simulink model "EvPowertrainController3EMDualFront"  (R2023a)
settings: configuration reference "VehicleFixed10ms" (kept outside this file)
model workspace (MAT data in the model file):
  CtrlVcuCnstrntPnltyFctr = 10000000
  CtrlVcuEMTrqSplitGrid = 200
  CtrlVcuPwrDeltaPnlty = 2
  CtrlVcuTracPwrErrPnlty = 6
  CtrlVcuTrqVecBrkThresh = 0.01
  CtrlVcuTrqVecIGain = 0
  CtrlVcuTrqVecMinTrq = 50
  CtrlVcuTrqVecPGain = -2000
  CtrlVcuTrqVecSteerThresh = 0.349065850399
  CtrlVcuTrqVecVelThresh = 2.5
undefined symbols (not defined in the file): CtrlVcuEvChrgLmtBpt, CtrlVcuEvRegenBrkCutOff, CtrlVcuEvRegenBrkSpdBpt, CtrlVcuEvSocBpt, eff, PlntBrkActrBoreFrnt, PlntBrkFrntBias, PlntBrkKinFricCffFrnt, PlntBrkNumPadsFrnt, PlntBrkPadMeanRadiusFrnt, PlntBrkPrsFctr, PlntBrkRearBias, PlntDiffrntl2Eff, PlntDiffrntl2Ratio, PlntDiffrntlEff, PlntDiffrntlRatio, PlntEM1EffTbl, PlntEM1Spd, PlntEM1Trq, PlntEM1TrqEff, PlntEM2EffTbl, PlntEM2Spd, PlntEM2Trq, PlntEM2TrqEff, PlntEM3EffTbl, PlntEM3Spd, PlntEM3Trq, PlntEM3TrqEff, PlntEMWhlGearEffFL, PlntEMWhlGearEffRL, PlntEMWhlGearRatioFL, PlntEMWhlGearRatioRL, PlntTransEffSpdBpt, PlntTransEffTbl, PlntTransEffTempBpt, PlntTransEffTrqBpt, PlntTransGearNumVect, PlntTransGearRatioVect, PlntVehDstCGFrntAxl, PlntVehDstCGRearAxl, PlntWhlLdRadius
libraries: simulink x13, autolibutils x2, slpidlib x2
(part 2 of 5)

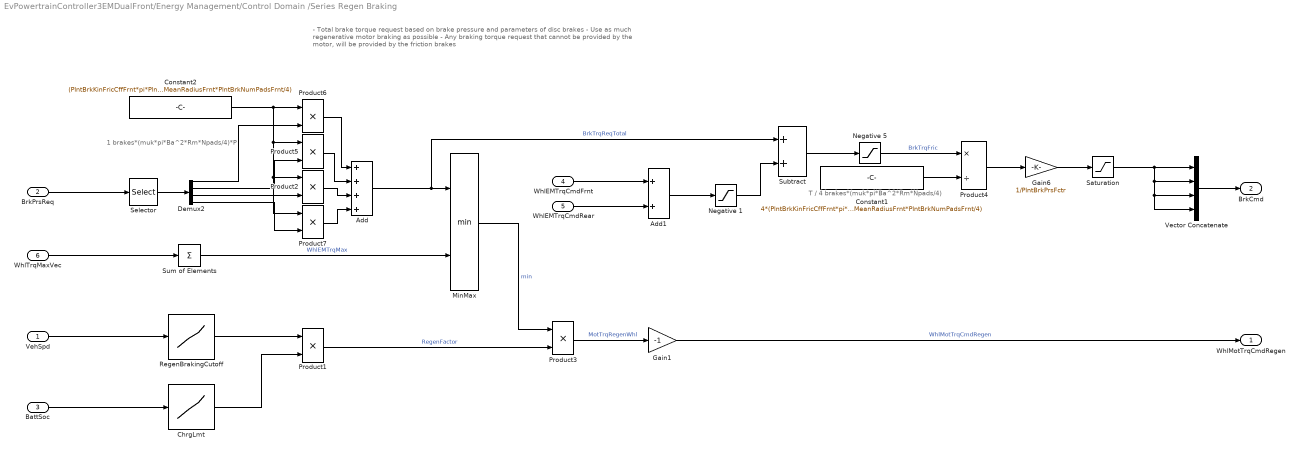
== system EvPowertrainController3EMDualFront/Energy Management/Control Domain /Series Regen Braking ==
  note: - Total brake torque request based on brake pressure and parameters of disc brakes
      | - Use as much regenerative motor braking as possible
      | - Any braking torque request that cannot be provided by the motor, will be provided by the friction brakes
  note: T / 4 brakes*(muk*pi*Ba^2*Rm*Npads/4)
  note: 1 brakes*(muk*pi*Ba^2*Rm*Npads/4)*P
  VehSpd : Inport
  "BrkPrsReq " : Inport  Port=2
  BattSoc : Inport  Port=3
  WhlEMTrqCmdFrnt : Inport  Port=4
  WhlEMTrqCmdRear : Inport  Port=5
  WhlTrqMaxVec : Inport  Port=6
  Add : Sum  Inputs=++++
  Add1 : Sum
  ChrgLmt : Lookup_n-D  NumberOfTableDimensions=1  BreakpointsForDimension1=CtrlVcuEvSocBpt  Table=CtrlVcuEvChrgLmtBpt  ExtrapMethod=Clip  UseLastTableValue=on  InternalRulePriority=Speed  RndMeth=Simplest
  Constant1 : Constant  Value=4*(PlntBrkKinFricCffFrnt*pi*PlntBrkActrBoreFrnt^2*PlntBrkPadMeanRadiusFrnt*PlntBrkNumPadsFrnt/4)
  Constant2 : Constant  Value=(PlntBrkKinFricCffFrnt*pi*PlntBrkActrBoreFrnt^2*PlntBrkPadMeanRadiusFrnt*PlntBrkNumPadsFrnt/4)
  Demux2 : Demux
  Gain1 : Gain  Gain=-1
  Gain6 : Gain  Gain=1/PlntBrkPrsFctr
  MinMax : MinMax  Inputs=2
  Negative 1 : Saturate  UpperLimit=0  LowerLimit=-inf
  Negative 5 : Saturate  UpperLimit=inf  LowerLimit=0
  Product{1..3,5..7} (6 alike) : Product
  Product4 : Product  Inputs=*/
  RegenBrakingCutoff : Lookup_n-D  NumberOfTableDimensions=1  BreakpointsForDimension1=CtrlVcuEvRegenBrkSpdBpt  Table=CtrlVcuEvRegenBrkCutOff  ExtrapMethod=Clip  UseLastTableValue=on  InternalRulePriority=Speed  RndMeth=Simplest
  Saturation : Saturate  UpperLimit=1  LowerLimit=0
  Selector : Selector  InputPortWidth=4  IndexOptions=Index vector (dialog)  Indices=[1 2 3 4]  OutputSizes=1
  Subtract : Sum
  Sum of Elements : Sum  Inputs=+
  Vector Concatenate : Concatenate  NumInputs=4
  " WhlMotTrqCmdRegen" : Outport  VectorParamsAs1DForOutWhenUnconnected=off
  " BrkCmd" : Outport  Port=2  VectorParamsAs1DForOutWhenUnconnected=off
  wires:
  Constant1/1 -> Product4/2
  MinMax/1 -> Product3/1  "min"
  ChrgLmt/1 -> Product1/2
  VehSpd/1 -> RegenBrakingCutoff/1
  RegenBrakingCutoff/1 -> Product1/1
  Product1/1 -> Product3/2  "RegenFactor"
  Subtract/1 -> Negative 5/1
  BattSoc/1 -> ChrgLmt/1
  Negative 5/1 -> Product4/1  "BrkTrqFric"
  Sum of Elements/1 -> MinMax/2  "WhlEMTrqMax"
  Demux2/2 -> Product5/2
  Demux2/1 -> Product6/2
  Selector/1 -> Demux2/1
  Product6/1 -> Add/1
  Product5/1 -> Add/2
  Add/1 -> Subtract/1, MinMax/1  "BrkTrqReqTotal"
  "BrkPrsReq "/1 -> Selector/1
  Vector Concatenate/1 -> " BrkCmd"/1
  Gain6/1 -> Saturation/1
  Product4/1 -> Gain6/1
  Saturation/1 -> Vector Concatenate/3, Vector Concatenate/4, Vector Concatenate/2, Vector Concatenate/1
  WhlTrqMaxVec/1 -> Sum of Elements/1
  Gain1/1 -> " WhlMotTrqCmdRegen"/1  "WhlMotTrqCmdRegen"
  Product3/1 -> Gain1/1  "MotTrqRegenWhl"
  Add1/1 -> Negative 1/1
  Negative 1/1 -> Subtract/2
  Product2/1 -> Add/3
  Product7/1 -> Add/4
  Demux2/3 -> Product2/2
  Demux2/4 -> Product7/2
  Constant2/1 -> Product7/1, Product2/1, Product5/1, Product6/1
  WhlEMTrqCmdFrnt/1 -> Add1/1
  WhlEMTrqCmdRear/1 -> Add1/2

== system EvPowertrainController3EMDualFront/Energy Management/Convert Whl to EMTrq Vector/2EM ==
  WhlEMTrqCmdFrnt : Inport
  WhlEMTrqCmdRear : Inport  Port=2
  EMAvgSpdVec : Inport  Port=3
  Diff Eta : Subsystem
  Diff Eta1 : Subsystem
  Divide1 : Product  Inputs=/*
  Divide2 : Product  Inputs=/*
  Gain1 : Gain  Gain=1/PlntDiffrntl2Ratio
  Gain3 : Gain  Gain=1/PlntDiffrntlRatio
  Selector : Selector  InputPortWidth=2  IndexOptions=Index vector (dialog)  Indices=[1]  OutputSizes=1
  Selector1 : Selector  InputPortWidth=2  IndexOptions=Index vector (dialog)  Indices=[2]  OutputSizes=1
  Unit Delay : UnitDelay  SampleTime=-1  HasFrameUpgradeWarning=on
  Unit Delay1 : UnitDelay  SampleTime=-1  HasFrameUpgradeWarning=on
  Vector Concatenate1 : Concatenate
  EMTrqCmd : Outport
  wires:
  WhlEMTrqCmdRear/1 -> Gain1/1
  Gain3/1 -> Divide2/2
  Divide2/1 -> Vector Concatenate1/1, Unit Delay/1
  WhlEMTrqCmdFrnt/1 -> Gain3/1
  Selector/1 -> Diff Eta/1(SpdIn)
  Unit Delay/1 -> Diff Eta/2(TrqIn)
  Diff Eta/1(eta) -> Divide2/1
  Diff Eta1/1(eta) -> Divide1/1
  Unit Delay1/1 -> Diff Eta1/2(TrqIn)
  Divide1/1 -> Unit Delay1/1, Vector Concatenate1/2
  Gain1/1 -> Divide1/2
  EMAvgSpdVec/1 -> Selector1/1, Selector/1
  Selector1/1 -> Diff Eta1/1(SpdIn)
  Vector Concatenate1/1 -> EMTrqCmd/1

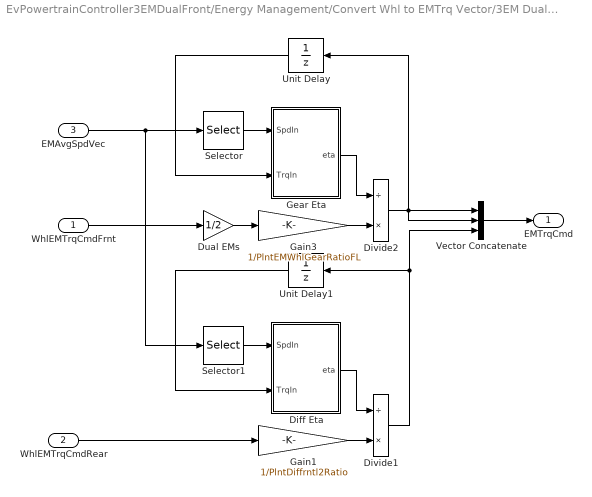
== system EvPowertrainController3EMDualFront/Energy Management/Convert Whl to EMTrq Vector/3EM Dual Front ==
  WhlEMTrqCmdFrnt : Inport
  WhlEMTrqCmdRear : Inport  Port=2
  EMAvgSpdVec : Inport  Port=3
  Diff Eta : Subsystem
  Divide1 : Product  Inputs=/*
  Divide2 : Product  Inputs=/*
  Dual EMs : Gain  Gain=1/2
  Gain1 : Gain  Gain=1/PlntDiffrntl2Ratio
  Gain3 : Gain  Gain=1/PlntEMWhlGearRatioFL
  Gear Eta : Subsystem
  Selector : Selector  InputPortWidth=2  IndexOptions=Index vector (dialog)  Indices=[1]  OutputSizes=1
  Selector1 : Selector  InputPortWidth=2  IndexOptions=Index vector (dialog)  Indices=[2]  OutputSizes=1
  Unit Delay : UnitDelay  SampleTime=-1  HasFrameUpgradeWarning=on
  Unit Delay1 : UnitDelay  SampleTime=-1  HasFrameUpgradeWarning=on
  Vector Concatenate : Concatenate  NumInputs=3
  EMTrqCmd : Outport
  wires:
  Selector1/1 -> Diff Eta/1(SpdIn)
  EMAvgSpdVec/1 -> Selector/1, Selector1/1
  Gain1/1 -> Divide1/2
  Unit Delay1/1 -> Diff Eta/2(TrqIn)
  Diff Eta/1(eta) -> Divide1/1
  Gear Eta/1(eta) -> Divide2/1
  Unit Delay/1 -> Gear Eta/2(TrqIn)
  Selector/1 -> Gear Eta/1(SpdIn)
  WhlEMTrqCmdFrnt/1 -> Dual EMs/1
  Gain3/1 -> Divide2/2
  WhlEMTrqCmdRear/1 -> Gain1/1
  Divide1/1 -> Vector Concatenate/3, Unit Delay1/1
  Vector Concatenate/1 -> EMTrqCmd/1
  Divide2/1 -> Vector Concatenate/1, Vector Concatenate/2, Unit Delay/1
  Dual EMs/1 -> Gain3/1

== system EvPowertrainController3EMDualFront/Energy Management/Convert Whl to EMTrq Vector/3EM Dual Rear ==
  WhlEMTrqCmdFrnt : Inport
  WhlEMTrqCmdRear : Inport  Port=2
  EMAvgSpdVec : Inport  Port=3
  Diff Eta : Subsystem
  Divide1 : Product  Inputs=/*
  Divide2 : Product  Inputs=/*
  Dual EMs : Gain  Gain=1/2
  Gain1 : Gain  Gain=1/PlntEMWhlGearRatioRL
  Gain3 : Gain  Gain=1/PlntDiffrntlRatio
  Gear Eta : Subsystem
  Selector : Selector  InputPortWidth=2  IndexOptions=Index vector (dialog)  Indices=[1]  OutputSizes=1
  Selector1 : Selector  InputPortWidth=2  IndexOptions=Index vector (dialog)  Indices=[2]  OutputSizes=1
  Unit Delay : UnitDelay  SampleTime=-1  HasFrameUpgradeWarning=on
  Unit Delay1 : UnitDelay  SampleTime=-1  HasFrameUpgradeWarning=on
  Vector Concatenate : Concatenate  NumInputs=3
  EMTrqCmd : Outport
  wires:
  WhlEMTrqCmdFrnt/1 -> Gain3/1
  Divide2/1 -> Unit Delay/1, Vector Concatenate/1
  Vector Concatenate/1 -> EMTrqCmd/1
  Divide1/1 -> Unit Delay1/1, Vector Concatenate/2, Vector Concatenate/3
  WhlEMTrqCmdRear/1 -> Dual EMs/1
  Gain3/1 -> Divide2/2
  Selector/1 -> Diff Eta/1(SpdIn)
  Unit Delay/1 -> Diff Eta/2(TrqIn)
  Diff Eta/1(eta) -> Divide2/1
  Gear Eta/1(eta) -> Divide1/1
  Unit Delay1/1 -> Gear Eta/2(TrqIn)
  Gain1/1 -> Divide1/2
  EMAvgSpdVec/1 -> Selector1/1, Selector/1
  Selector1/1 -> Gear Eta/1(SpdIn)
  Dual EMs/1 -> Gain1/1

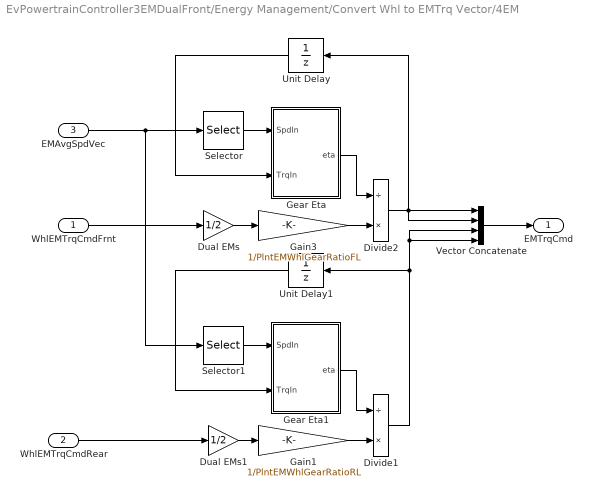
== system EvPowertrainController3EMDualFront/Energy Management/Convert Whl to EMTrq Vector/4EM ==
  WhlEMTrqCmdFrnt : Inport
  WhlEMTrqCmdRear : Inport  Port=2
  EMAvgSpdVec : Inport  Port=3
  Divide1 : Product  Inputs=/*
  Divide2 : Product  Inputs=/*
  Dual EMs : Gain  Gain=1/2
  Dual EMs1 : Gain  Gain=1/2
  Gain1 : Gain  Gain=1/PlntEMWhlGearRatioRL
  Gain3 : Gain  Gain=1/PlntEMWhlGearRatioFL
  Gear Eta : Subsystem
  Gear Eta1 : Subsystem
  Selector : Selector  InputPortWidth=2  IndexOptions=Index vector (dialog)  Indices=[1]  OutputSizes=1
  Selector1 : Selector  InputPortWidth=2  IndexOptions=Index vector (dialog)  Indices=[2]  OutputSizes=1
  Unit Delay : UnitDelay  SampleTime=-1  HasFrameUpgradeWarning=on
  Unit Delay1 : UnitDelay  SampleTime=-1  HasFrameUpgradeWarning=on
  Vector Concatenate : Concatenate  NumInputs=4
  EMTrqCmd : Outport
  wires:
  Dual EMs1/1 -> Gain1/1
  Selector1/1 -> Gear Eta1/1(SpdIn)
  EMAvgSpdVec/1 -> Selector/1, Selector1/1
  Gain1/1 -> Divide1/2
  Unit Delay1/1 -> Gear Eta1/2(TrqIn)
  Gear Eta1/1(eta) -> Divide1/1
  Gear Eta/1(eta) -> Divide2/1
  Unit Delay/1 -> Gear Eta/2(TrqIn)
  Selector/1 -> Gear Eta/1(SpdIn)
  Gain3/1 -> Divide2/2
  WhlEMTrqCmdRear/1 -> Dual EMs1/1
  Divide1/1 -> Vector Concatenate/4, Vector Concatenate/3, Unit Delay1/1
  Vector Concatenate/1 -> EMTrqCmd/1
  Divide2/1 -> Vector Concatenate/2, Unit Delay/1, Vector Concatenate/1
  WhlEMTrqCmdFrnt/1 -> Dual EMs/1
  Dual EMs/1 -> Gain3/1

== system EvPowertrainController3EMDualFront/Energy Management/Hamiltonian computation and minimization/Pwr Rate Limit ==
  note: There could be instances where an mot trq command produces the minimum cost, but differs greatly from the previously selected mot trq.
      |
      | This function will calculate the difference in power between the current mot power vector and the previously selected mot pwr.  This term is added to the total cost function, and will help limit the rate at which the mot power (and torque) can change from time step to time step.
  note: Alternative to using
      | abs funciton
  WhlEMTrqFVec : Inport
  WhlSpd : Inport  Port=2
  PrevWhlEMTrqCmdF : Inport  Port=3
  Product1 : Product
  Product6 : Product
  Product7 : Product
  PwrDelta Penalty : Gain  Gain=CtrlVcuPwrDeltaPnlty
  Sqrt1 : Sqrt
  Subtract : Sum  Inputs=+-
  W2kW : Gain  Gain=1/1000
  EMPwrDelta : Outport  VectorParamsAs1DForOutWhenUnconnected=off
  wires:
  Product7/1 -> Sqrt1/1
  Product6/1 -> Subtract/1  "PwrVec"
  Product1/1 -> Subtract/2  "PrevPwr"
  WhlSpd/1 -> Product6/2, Product1/1
  PrevWhlEMTrqCmdF/1 -> Product1/2
  Subtract/1 -> Product7/1, Product7/2
  Sqrt1/1 -> W2kW/1
  WhlEMTrqFVec/1 -> Product6/1
  W2kW/1 -> PwrDelta Penalty/1
  PwrDelta Penalty/1 -> EMPwrDelta/1

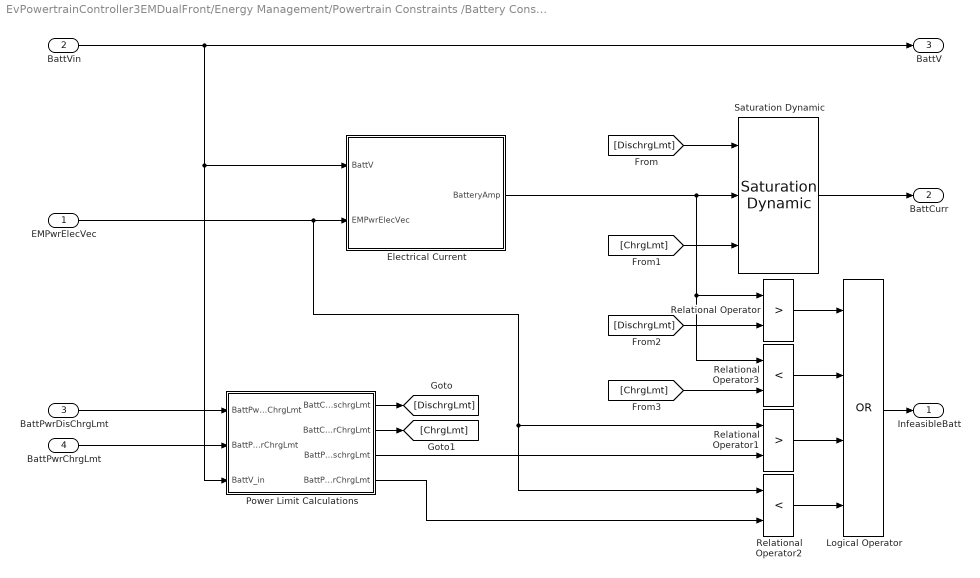
== system EvPowertrainController3EMDualFront/Energy Management/Powertrain Constraints /Battery Constraint ==
  EMPwrElecVec : Inport
  BattVin : Inport  Port=2
  BattPwrDisChrgLmt : Inport  Port=3
  "BattPwrChrgLmt " : Inport  Port=4
  Electrical Current : Subsystem
  Logical Operator : Logic  Operator=OR  Inputs=4  AllPortsSameDT=off  OutDataTypeStr=boolean
  Power Limit Calculations : Subsystem
  Relational Operator : RelationalOperator  Operator=>  OutDataTypeStr=boolean  InputSameDT=off
  Relational Operator1 : RelationalOperator  Operator=>  OutDataTypeStr=boolean  InputSameDT=off
  Relational Operator2 : RelationalOperator  Operator=<  OutDataTypeStr=boolean  InputSameDT=off
  Relational Operator3 : RelationalOperator  Operator=<  OutDataTypeStr=boolean  InputSameDT=off
  Saturation Dynamic : simulink/Discontinuities/Saturation Dynamic  OutMin=[]  OutMax=[]  OutDataTypeStr=Inherit: Same as second input  OutDataType=fixdt(1, 16)  OutScaling=2^-10  DoSatur=off
  InfeasibleBatt : Outport  VectorParamsAs1DForOutWhenUnconnected=off
  BattCurr : Outport  Port=2  VectorParamsAs1DForOutWhenUnconnected=off
  BattV : Outport  Port=3  VectorParamsAs1DForOutWhenUnconnected=off
  wires:
  Saturation Dynamic/1 -> BattCurr/1
  Logical Operator/1 -> InfeasibleBatt/1
  Relational Operator1/1 -> Logical Operator/3
  EMPwrElecVec/1 -> Relational Operator1/1, Relational Operator2/1, Electrical Current/2(EMPwrElecVec)
  Relational Operator2/1 -> Logical Operator/4
  Power Limit Calculations/3(BattPwrDischrgLmt) -> Relational Operator1/2
  Power Limit Calculations/4(BattPwrChrgLmt) -> Relational Operator2/2
  BattVin/1 -> Electrical Current/1(BattV), Power Limit Calculations/3(BattV_in), BattV/1
  [DischrgLmt] -> Saturation Dynamic/1
  [ChrgLmt] -> Saturation Dynamic/3
  Relational Operator/1 -> Logical Operator/1
  Electrical Current/1(BatteryAmp) -> Relational Operator3/1, Relational Operator/1, Saturation Dynamic/2
  "BattPwrChrgLmt "/1 -> Power Limit Calculations/2("BattPwrChrgLmt ")
  BattPwrDisChrgLmt/1 -> Power Limit Calculations/1(BattPwrDisChrgLmt)
  Power Limit Calculations/1(BattCurrDischrgLmt) -> [DischrgLmt]
  Power Limit Calculations/2(BattCurrChrgLmt) -> [ChrgLmt]
  [DischrgLmt] -> Relational Operator/2
  [ChrgLmt] -> Relational Operator3/2
  Relational Operator3/1 -> Logical Operator/2

== system EvPowertrainController3EMDualFront/Energy Management/Powertrain Constraints /EM Constraint Front ==
  WhlTrqCmd : Inport
  EMAvgSpdVec : Inport  Port=2
  WhlEMTrqSplitVecFrnt : Inport  Port=3
  WhlTrqMaxVec : Inport  Port=4
  Maximum Torque : Subsystem  VariantControl=2EM
  Tabular Power Loss Data : Subsystem  Variant=on  VariantControlMode=label  VariantControl=Choice  LabelModeActiveChoice=3EM Dual Front or 4EM
  WhlEMTrqSatVec : Outport  VectorParamsAs1DForOutWhenUnconnected=off
  InfeasibleEMVec : Outport  Port=2  VectorParamsAs1DForOutWhenUnconnected=off
  EMPwrElecVec : Outport  Port=3  VectorParamsAs1DForOutWhenUnconnected=off
  wires:
  WhlTrqMaxVec/1 -> Maximum Torque/3(WhlTrqMaxVec)
  Tabular Power Loss Data/1(EMPwrElecVec) -> EMPwrElecVec/1
  Maximum Torque/2(InfeasibleEMVec) -> InfeasibleEMVec/1
  WhlEMTrqSplitVecFrnt/1 -> Maximum Torque/2(WhlEMTrqSplitVecFrnt)
  WhlTrqCmd/1 -> Maximum Torque/1(WhlTrqCmd)
  EMAvgSpdVec/1 -> Tabular Power Loss Data/1(EMAvgSpdVec)
  Maximum Torque/1(WhlEMTrqSatVec) -> Tabular Power Loss Data/2(WhlEMTrqSatVec), WhlEMTrqSatVec/1

== system EvPowertrainController3EMDualFront/Energy Management/Powertrain Constraints /EM Constraint Rear ==
  WhlTrqCmd : Inport
  EMAvgSpdVec : Inport  Port=2
  WhlEMTrqSplitVecRear : Inport  Port=3
  WhlTrqMaxVec : Inport  Port=4
  Maximum Torque : Subsystem  VariantControl=2EM
  Tabular Power Loss Data : Subsystem  Variant=on  VariantControlMode=label  VariantControl=Choice  LabelModeActiveChoice=3EM Dual Front
  WhlEMTrqSatVec : Outport  VectorParamsAs1DForOutWhenUnconnected=off
  InfeasibleEMVec : Outport  Port=2  VectorParamsAs1DForOutWhenUnconnected=off
  EMPwrElecVec : Outport  Port=3  VectorParamsAs1DForOutWhenUnconnected=off
  wires:
  Maximum Torque/1(WhlEMTrqSatVec) -> WhlEMTrqSatVec/1, Tabular Power Loss Data/2(WhlEMTrqSatVec)
  EMAvgSpdVec/1 -> Tabular Power Loss Data/1(EMAvgSpdVec)
  WhlTrqCmd/1 -> Maximum Torque/1(WhlTrqCmd)
  WhlEMTrqSplitVecRear/1 -> Maximum Torque/2(WhlEMTrqSplitVecRear)
  Maximum Torque/2(InfeasibleEMVec) -> InfeasibleEMVec/1
  Tabular Power Loss Data/1(EMPwrElecVec) -> EMPwrElecVec/1
  WhlTrqMaxVec/1 -> Maximum Torque/3(WhlTrqMaxVec)

== system EvPowertrainController3EMDualFront/Torque Vectoring/3EM/Create EMTrq Vector ==
  EMTrqSplit : Inport
  EMTrqCmd : Inport  Port=2
  3EMDualFront : Subsystem  VariantControl=3EMDualFront
  3EMDualRear : Subsystem  VariantControl=3EMDualRear
  EMTrqCmdFinal : Outport

== system EvPowertrainController3EMDualFront/Torque Vectoring/3EM/EMTrq ==
  EMSpd : Inport
  EMTrqCmd : Inport  Port=2
  3EMDualFront : Subsystem  VariantControl=3EMDualFront
  3EMDualRear : Subsystem  VariantControl=3EMDualRear
  EMTrqMax : Outport
  EMTrqL : Outport  Port=2
  EMTrqR : Outport  Port=3

== system EvPowertrainController3EMDualFront/Torque Vectoring/4EM/EMTrq ==
  EMSpd : Inport
  EMTrqCmd : Inport  Port=2
  Dual Front : Subsystem  VariantControl=3EMDualFront
  Dual Rear : Subsystem  VariantControl=3EMDualRear
  EMTrqMaxFrnt : Outport
  EMTrqFL : Outport  Port=2
  EMTrqFR : Outport  Port=3
  EMTrqMaxRear : Outport  Port=4
  EMTrqRL : Outport  Port=5
  EMTrqRR : Outport  Port=6
  wires:
  EMTrqCmd/1 -> Dual Rear/2(EMTrqCmd), Dual Front/2(EMTrqCmd)
  Dual Front/1(EMTrqMaxFrnt) -> EMTrqMaxFrnt/1
  EMSpd/1 -> Dual Rear/1(EMSpd), Dual Front/1(EMSpd)
  Dual Rear/1(EMTrqMaxRear) -> EMTrqMaxRear/1
  Dual Front/3(EMTrqFR) -> EMTrqFR/1
  Dual Front/2(EMTrqFL) -> EMTrqFL/1
  Dual Rear/3(EMTrqRR) -> EMTrqRR/1
  Dual Rear/2(EMTrqRL) -> EMTrqRL/1

== system EvPowertrainController3EMDualFront/Accel Pedal to Traction Wheel Torque Request/EM2WhlTrq/2EM/EMTrq2WhlTrqFrnt ==
  Gear : Inport
  EMTrqCmd : Inport  Port=2
  EMSpd : Inport  Port=3
  No Transmission : Subsystem  VariantControl=3
  Transmission : Subsystem  VariantControl=1
  WhlMotTrq : Outport

== system EvPowertrainController3EMDualFront/Accel Pedal to Traction Wheel Torque Request/EM2WhlTrq/2EM/EMTrq2WhlTrqRear ==
  Gear : Inport
  EMTrqCmd : Inport  Port=2
  EMSpd : Inport  Port=3
  No Transmission : Subsystem  VariantControl=3
  Transmission : Subsystem  VariantControl=1
  WhlMotTrq : Outport

== system EvPowertrainController3EMDualFront/Accel Pedal to Traction Wheel Torque Request/EM2WhlTrq/2EM/Maximum Torque Front Axle ==
  EMSpd : Inport
  MaxEMTrqVsSpd : Lookup_n-D  NumberOfTableDimensions=1  BreakpointsForDimension1=PlntEM1Spd  Table=PlntEM1Trq  ExtrapMethod=Clip  UseLastTableValue=on  InternalRulePriority=Speed  OutDataTypeStr=Inherit: Inherit from 'Table data'  RndMeth=Simplest
  EMTrq : Outport  VectorParamsAs1DForOutWhenUnconnected=off
  wires:
  MaxEMTrqVsSpd/1 -> EMTrq/1
  EMSpd/1 -> MaxEMTrqVsSpd/1

== system EvPowertrainController3EMDualFront/Accel Pedal to Traction Wheel Torque Request/EM2WhlTrq/2EM/Maximum Torque Rear Axle ==
  EMSpd : Inport
  MaxEMTrqVsSpd : Lookup_n-D  NumberOfTableDimensions=1  BreakpointsForDimension1=PlntEM2Spd  Table=PlntEM2Trq  ExtrapMethod=Clip  UseLastTableValue=on  InternalRulePriority=Speed  OutDataTypeStr=Inherit: Inherit from 'Table data'  RndMeth=Simplest
  EMTrq : Outport  VectorParamsAs1DForOutWhenUnconnected=off
  wires:
  MaxEMTrqVsSpd/1 -> EMTrq/1
  EMSpd/1 -> MaxEMTrqVsSpd/1

== system EvPowertrainController3EMDualFront/Accel Pedal to Traction Wheel Torque Request/EM2WhlTrq/2EM/VehSpd2EMSpd ==
  Gear : Inport
  VehSpd : Inport  Port=2
  No Transmission : Subsystem  VariantControl=3
  Transmission : Subsystem  VariantControl=1
  EMSpdFrntAxl : Outport
  EMSpdRearAxl : Outport  Port=2

== system EvPowertrainController3EMDualFront/Accel Pedal to Traction Wheel Torque Request/EM2WhlTrq/3EM Dual Front/EMTrq2WhlTrqFrnt ==
  Gear : Inport
  EMTrqCmd : Inport  Port=2
  EMSpd : Inport  Port=3
  No Transmission : Subsystem  VariantControl=3
  Transmission : Subsystem  VariantControl=1
  WhlMotTrq : Outport

== system EvPowertrainController3EMDualFront/Accel Pedal to Traction Wheel Torque Request/EM2WhlTrq/3EM Dual Front/EMTrq2WhlTrqRear ==
  Gear : Inport
  EMTrqCmd : Inport  Port=2
  EMSpd : Inport  Port=3
  No Transmission : Subsystem  VariantControl=3
  Transmission : Subsystem  VariantControl=1
  WhlMotTrq : Outport

== system EvPowertrainController3EMDualFront/Accel Pedal to Traction Wheel Torque Request/EM2WhlTrq/3EM Dual Front/Maximum Torque Front Axle ==
  EMSpd : Inport
  MaxEMTrqVsSpd : Lookup_n-D  NumberOfTableDimensions=1  BreakpointsForDimension1=PlntEM1Spd  Table=PlntEM1Trq  ExtrapMethod=Clip  UseLastTableValue=on  InternalRulePriority=Speed  OutDataTypeStr=Inherit: Inherit from 'Table data'  RndMeth=Simplest
  EMTrq : Outport  VectorParamsAs1DForOutWhenUnconnected=off
  wires:
  EMSpd/1 -> MaxEMTrqVsSpd/1
  MaxEMTrqVsSpd/1 -> EMTrq/1

== system EvPowertrainController3EMDualFront/Accel Pedal to Traction Wheel Torque Request/EM2WhlTrq/3EM Dual Front/Maximum Torque Rear Axle ==
  EMSpd : Inport
  MaxEMTrqVsSpd : Lookup_n-D  NumberOfTableDimensions=1  BreakpointsForDimension1=PlntEM3Spd  Table=PlntEM3Trq  ExtrapMethod=Clip  UseLastTableValue=on  InternalRulePriority=Speed  OutDataTypeStr=Inherit: Inherit from 'Table data'  RndMeth=Simplest
  EMTrq : Outport  VectorParamsAs1DForOutWhenUnconnected=off
  wires:
  EMSpd/1 -> MaxEMTrqVsSpd/1
  MaxEMTrqVsSpd/1 -> EMTrq/1

== system EvPowertrainController3EMDualFront/Accel Pedal to Traction Wheel Torque Request/EM2WhlTrq/3EM Dual Front/VehSpd2EMSpd ==
  Gear : Inport
  VehSpd : Inport  Port=2
  No Transmission : Subsystem  VariantControl=3
  Transmission : Subsystem  VariantControl=1
  EMSpdFrntAxl : Outport
  EMSpdRearAxl : Outport  Port=2

== system EvPowertrainController3EMDualFront/Accel Pedal to Traction Wheel Torque Request/EM2WhlTrq/3EM Dual Rear/EMTrq2WhlTrqFrnt ==
  Gear : Inport
  EMTrqCmd : Inport  Port=2
  EMSpd : Inport  Port=3
  No Transmission : Subsystem  VariantControl=3
  Transmission : Subsystem  VariantControl=1
  WhlMotTrq : Outport

== system EvPowertrainController3EMDualFront/Accel Pedal to Traction Wheel Torque Request/EM2WhlTrq/3EM Dual Rear/EMTrq2WhlTrqRear ==
  Gear : Inport
  EMTrqCmd : Inport  Port=2
  EMSpd : Inport  Port=3
  No Transmission : Subsystem  VariantControl=3
  Transmission : Subsystem  VariantControl=1
  WhlMotTrq : Outport

== system EvPowertrainController3EMDualFront/Accel Pedal to Traction Wheel Torque Request/EM2WhlTrq/3EM Dual Rear/Maximum Torque Front Axle ==
  EMSpd : Inport
  MaxEMTrqVsSpd : Lookup_n-D  NumberOfTableDimensions=1  BreakpointsForDimension1=PlntEM1Spd  Table=PlntEM1Trq  ExtrapMethod=Clip  UseLastTableValue=on  InternalRulePriority=Speed  OutDataTypeStr=Inherit: Inherit from 'Table data'  RndMeth=Simplest
  EMTrq : Outport  VectorParamsAs1DForOutWhenUnconnected=off
  wires:
  MaxEMTrqVsSpd/1 -> EMTrq/1
  EMSpd/1 -> MaxEMTrqVsSpd/1

== system EvPowertrainController3EMDualFront/Accel Pedal to Traction Wheel Torque Request/EM2WhlTrq/3EM Dual Rear/Maximum Torque Rear Axle ==
  EMSpd : Inport
  MaxEMTrqVsSpd : Lookup_n-D  NumberOfTableDimensions=1  BreakpointsForDimension1=PlntEM3Spd  Table=PlntEM3Trq  ExtrapMethod=Clip  UseLastTableValue=on  InternalRulePriority=Speed  OutDataTypeStr=Inherit: Inherit from 'Table data'  RndMeth=Simplest
  EMTrq : Outport  VectorParamsAs1DForOutWhenUnconnected=off
  wires:
  EMSpd/1 -> MaxEMTrqVsSpd/1
  MaxEMTrqVsSpd/1 -> EMTrq/1

== system EvPowertrainController3EMDualFront/Accel Pedal to Traction Wheel Torque Request/EM2WhlTrq/3EM Dual Rear/VehSpd2EMSpd ==
  Gear : Inport
  VehSpd : Inport  Port=2
  No Transmission : Subsystem  VariantControl=3
  Transmission : Subsystem  VariantControl=1
  EMSpdFrntAxl : Outport
  EMSpdRearAxl : Outport  Port=2

== system EvPowertrainController3EMDualFront/Accel Pedal to Traction Wheel Torque Request/EM2WhlTrq/4EM/EMTrq2WhlTrqFrnt ==
  Gear : Inport
  EMTrqCmd : Inport  Port=2
  EMSpd : Inport  Port=3
  No Transmission : Subsystem  VariantControl=3
  Transmission : Subsystem  VariantControl=1
  WhlMotTrq : Outport

== system EvPowertrainController3EMDualFront/Accel Pedal to Traction Wheel Torque Request/EM2WhlTrq/4EM/EMTrq2WhlTrqRear ==
  Gear : Inport
  EMTrqCmd : Inport  Port=2
  EMSpd : Inport  Port=3
  No Transmission : Subsystem  VariantControl=3
  Transmission : Subsystem  VariantControl=1
  WhlMotTrq : Outport

== system EvPowertrainController3EMDualFront/Accel Pedal to Traction Wheel Torque Request/EM2WhlTrq/4EM/Maximum Torque Front Axle ==
  EMSpd : Inport
  MaxEMTrqVsSpd : Lookup_n-D  NumberOfTableDimensions=1  BreakpointsForDimension1=PlntEM1Spd  Table=PlntEM1Trq  ExtrapMethod=Clip  UseLastTableValue=on  InternalRulePriority=Speed  OutDataTypeStr=Inherit: Inherit from 'Table data'  RndMeth=Simplest
  EMTrq : Outport  VectorParamsAs1DForOutWhenUnconnected=off
  wires:
  EMSpd/1 -> MaxEMTrqVsSpd/1
  MaxEMTrqVsSpd/1 -> EMTrq/1

== system EvPowertrainController3EMDualFront/Accel Pedal to Traction Wheel Torque Request/EM2WhlTrq/4EM/Maximum Torque Rear Axle ==
  EMSpd : Inport
  MaxEMTrqVsSpd : Lookup_n-D  NumberOfTableDimensions=1  BreakpointsForDimension1=PlntEM3Spd  Table=PlntEM3Trq  ExtrapMethod=Clip  UseLastTableValue=on  InternalRulePriority=Speed  OutDataTypeStr=Inherit: Inherit from 'Table data'  RndMeth=Simplest
  EMTrq : Outport  VectorParamsAs1DForOutWhenUnconnected=off
  wires:
  MaxEMTrqVsSpd/1 -> EMTrq/1
  EMSpd/1 -> MaxEMTrqVsSpd/1

== system EvPowertrainController3EMDualFront/Accel Pedal to Traction Wheel Torque Request/EM2WhlTrq/4EM/VehSpd2EMSpd ==
  Gear : Inport
  VehSpd : Inport  Port=2
  No Transmission : Subsystem  VariantControl=3
  Transmission : Subsystem  VariantControl=1
  EMSpdFrntAxl : Outport
  EMSpdRearAxl : Outport  Port=2

== system EvPowertrainController3EMDualFront/Energy Management/Calculate Average EMSpd and Wheel Torque Curves for Front and Rear Axles/2EM/EMTrq2WhlTrqFrnt ==
  Gear : Inport
  EMTrqCmd : Inport  Port=2
  EMSpd : Inport  Port=3
  No Transmission : Subsystem  VariantControl=3
  Transmission : Subsystem  VariantControl=1
  WhlMotTrq : Outport

== system EvPowertrainController3EMDualFront/Energy Management/Calculate Average EMSpd and Wheel Torque Curves for Front and Rear Axles/2EM/EMTrq2WhlTrqRear ==
  Gear : Inport
  EMTrqCmd : Inport  Port=2
  EMSpd : Inport  Port=3
  No Transmission : Subsystem  VariantControl=3
  Transmission : Subsystem  VariantControl=1
  WhlMotTrq : Outport

== system EvPowertrainController3EMDualFront/Energy Management/Calculate Average EMSpd and Wheel Torque Curves for Front and Rear Axles/2EM/Maximum Torque Front Axle ==
  EMSpd : Inport
  MaxEMTrqVsSpd : Lookup_n-D  NumberOfTableDimensions=1  BreakpointsForDimension1=PlntEM1Spd  Table=PlntEM1Trq  ExtrapMethod=Clip  UseLastTableValue=on  InternalRulePriority=Speed  OutDataTypeStr=Inherit: Inherit from 'Table data'  RndMeth=Simplest
  EMTrq : Outport  VectorParamsAs1DForOutWhenUnconnected=off
  wires:
  MaxEMTrqVsSpd/1 -> EMTrq/1
  EMSpd/1 -> MaxEMTrqVsSpd/1

== system EvPowertrainController3EMDualFront/Energy Management/Calculate Average EMSpd and Wheel Torque Curves for Front and Rear Axles/2EM/Maximum Torque Rear Axle ==
  EMSpd : Inport
  MaxEMTrqVsSpd : Lookup_n-D  NumberOfTableDimensions=1  BreakpointsForDimension1=PlntEM2Spd  Table=PlntEM2Trq  ExtrapMethod=Clip  UseLastTableValue=on  InternalRulePriority=Speed  OutDataTypeStr=Inherit: Inherit from 'Table data'  RndMeth=Simplest
  EMTrq : Outport  VectorParamsAs1DForOutWhenUnconnected=off
  wires:
  MaxEMTrqVsSpd/1 -> EMTrq/1
  EMSpd/1 -> MaxEMTrqVsSpd/1

== system EvPowertrainController3EMDualFront/Energy Management/Calculate Average EMSpd and Wheel Torque Curves for Front and Rear Axles/3EM Dual Front/EMTrq2WhlTrqFrnt ==
  Gear : Inport
  EMTrqCmd : Inport  Port=2
  EMSpd : Inport  Port=3
  No Transmission : Subsystem  VariantControl=3
  Transmission : Subsystem  VariantControl=1
  WhlMotTrq : Outport

== system EvPowertrainController3EMDualFront/Energy Management/Calculate Average EMSpd and Wheel Torque Curves for Front and Rear Axles/3EM Dual Front/EMTrq2WhlTrqRear ==
  Gear : Inport
  EMTrqCmd : Inport  Port=2
  EMSpd : Inport  Port=3
  No Transmission : Subsystem  VariantControl=3
  Transmission : Subsystem  VariantControl=1
  WhlMotTrq : Outport

== system EvPowertrainController3EMDualFront/Energy Management/Calculate Average EMSpd and Wheel Torque Curves for Front and Rear Axles/3EM Dual Front/Maximum Torque Front Axle ==
  EMSpd : Inport
  MaxEMTrqVsSpd : Lookup_n-D  NumberOfTableDimensions=1  BreakpointsForDimension1=PlntEM1Spd  Table=PlntEM1Trq  ExtrapMethod=Clip  UseLastTableValue=on  InternalRulePriority=Speed  OutDataTypeStr=Inherit: Inherit from 'Table data'  RndMeth=Simplest
  EMTrq : Outport  VectorParamsAs1DForOutWhenUnconnected=off
  wires:
  EMSpd/1 -> MaxEMTrqVsSpd/1
  MaxEMTrqVsSpd/1 -> EMTrq/1

== system EvPowertrainController3EMDualFront/Energy Management/Calculate Average EMSpd and Wheel Torque Curves for Front and Rear Axles/3EM Dual Front/Maximum Torque Rear Axle ==
  EMSpd : Inport
  MaxEMTrqVsSpd : Lookup_n-D  NumberOfTableDimensions=1  BreakpointsForDimension1=PlntEM3Spd  Table=PlntEM3Trq  ExtrapMethod=Clip  UseLastTableValue=on  InternalRulePriority=Speed  OutDataTypeStr=Inherit: Inherit from 'Table data'  RndMeth=Simplest
  EMTrq : Outport  VectorParamsAs1DForOutWhenUnconnected=off
  wires:
  EMSpd/1 -> MaxEMTrqVsSpd/1
  MaxEMTrqVsSpd/1 -> EMTrq/1

== system EvPowertrainController3EMDualFront/Energy Management/Calculate Average EMSpd and Wheel Torque Curves for Front and Rear Axles/3EM Dual Rear/EMTrq2WhlTrqFrnt ==
  Gear : Inport
  EMTrqCmd : Inport  Port=2
  EMSpd : Inport  Port=3
  No Transmission : Subsystem  VariantControl=3
  Transmission : Subsystem  VariantControl=1
  WhlMotTrq : Outport

== system EvPowertrainController3EMDualFront/Energy Management/Calculate Average EMSpd and Wheel Torque Curves for Front and Rear Axles/3EM Dual Rear/EMTrq2WhlTrqRear ==
  Gear : Inport
  EMTrqCmd : Inport  Port=2
  EMSpd : Inport  Port=3
  No Transmission : Subsystem  VariantControl=3
  Transmission : Subsystem  VariantControl=1
  WhlMotTrq : Outport

== system EvPowertrainController3EMDualFront/Energy Management/Calculate Average EMSpd and Wheel Torque Curves for Front and Rear Axles/3EM Dual Rear/Maximum Torque Front Axle ==
  EMSpd : Inport
  MaxEMTrqVsSpd : Lookup_n-D  NumberOfTableDimensions=1  BreakpointsForDimension1=PlntEM1Spd  Table=PlntEM1Trq  ExtrapMethod=Clip  UseLastTableValue=on  InternalRulePriority=Speed  OutDataTypeStr=Inherit: Inherit from 'Table data'  RndMeth=Simplest
  EMTrq : Outport  VectorParamsAs1DForOutWhenUnconnected=off
  wires:
  MaxEMTrqVsSpd/1 -> EMTrq/1
  EMSpd/1 -> MaxEMTrqVsSpd/1

== system EvPowertrainController3EMDualFront/Energy Management/Calculate Average EMSpd and Wheel Torque Curves for Front and Rear Axles/3EM Dual Rear/Maximum Torque Rear Axle ==
  EMSpd : Inport
  MaxEMTrqVsSpd : Lookup_n-D  NumberOfTableDimensions=1  BreakpointsForDimension1=PlntEM3Spd  Table=PlntEM3Trq  ExtrapMethod=Clip  UseLastTableValue=on  InternalRulePriority=Speed  OutDataTypeStr=Inherit: Inherit from 'Table data'  RndMeth=Simplest
  EMTrq : Outport  VectorParamsAs1DForOutWhenUnconnected=off
  wires:
  EMSpd/1 -> MaxEMTrqVsSpd/1
  MaxEMTrqVsSpd/1 -> EMTrq/1

== system EvPowertrainController3EMDualFront/Energy Management/Calculate Average EMSpd and Wheel Torque Curves for Front and Rear Axles/4EM/EMTrq2WhlTrqFrnt ==
  Gear : Inport
  EMTrqCmd : Inport  Port=2
  EMSpd : Inport  Port=3
  No Transmission : Subsystem  VariantControl=3
  Transmission : Subsystem  VariantControl=1
  WhlMotTrq : Outport

== system EvPowertrainController3EMDualFront/Energy Management/Calculate Average EMSpd and Wheel Torque Curves for Front and Rear Axles/4EM/EMTrq2WhlTrqRear ==
  Gear : Inport
  EMTrqCmd : Inport  Port=2
  EMSpd : Inport  Port=3
  No Transmission : Subsystem  VariantControl=3
  Transmission : Subsystem  VariantControl=1
  WhlMotTrq : Outport

== system EvPowertrainController3EMDualFront/Energy Management/Calculate Average EMSpd and Wheel Torque Curves for Front and Rear Axles/4EM/Maximum Torque Front Axle ==
  EMSpd : Inport
  MaxEMTrqVsSpd : Lookup_n-D  NumberOfTableDimensions=1  BreakpointsForDimension1=PlntEM1Spd  Table=PlntEM1Trq  ExtrapMethod=Clip  UseLastTableValue=on  InternalRulePriority=Speed  OutDataTypeStr=Inherit: Inherit from 'Table data'  RndMeth=Simplest
  EMTrq : Outport  VectorParamsAs1DForOutWhenUnconnected=off
  wires:
  EMSpd/1 -> MaxEMTrqVsSpd/1
  MaxEMTrqVsSpd/1 -> EMTrq/1

== system EvPowertrainController3EMDualFront/Energy Management/Calculate Average EMSpd and Wheel Torque Curves for Front and Rear Axles/4EM/Maximum Torque Rear Axle ==
  EMSpd : Inport
  MaxEMTrqVsSpd : Lookup_n-D  NumberOfTableDimensions=1  BreakpointsForDimension1=PlntEM3Spd  Table=PlntEM3Trq  ExtrapMethod=Clip  UseLastTableValue=on  InternalRulePriority=Speed  OutDataTypeStr=Inherit: Inherit from 'Table data'  RndMeth=Simplest
  EMTrq : Outport  VectorParamsAs1DForOutWhenUnconnected=off
  wires:
  MaxEMTrqVsSpd/1 -> EMTrq/1
  EMSpd/1 -> MaxEMTrqVsSpd/1

== system EvPowertrainController3EMDualFront/Energy Management/Control Domain /Rear Axle EM Torque Vector/2EM or 3EM Dual Front ==
  EMAvgSpdVec : Inport
  Diff Eta : Subsystem
  Divide2 : Product  Inputs=**
  EMTrq Control Vector Traction : Constant  Value=linspace(0, max(PlntEM2Trq), CtrlVcuEMTrqSplitGrid)  SampleTime=-1
  Gain : Gain  Gain=-1
  Gain3 : Gain  Gain=PlntDiffrntl2Ratio
  Selector : Selector  InputPortWidth=2  IndexOptions=Index vector (dialog)  Indices=[2]  OutputSizes=1
  WhlEMRearVecPos : Outport
  WhlEMRearVecNeg : Outport  Port=2
  wires:
  Gain/1 -> WhlEMRearVecNeg/1
  EMAvgSpdVec/1 -> Selector/1
  EMTrq Control Vector Traction/1 -> Diff Eta/2(TrqIn), Gain3/1
  Divide2/1 -> Gain/1, WhlEMRearVecPos/1
  Diff Eta/1(eta) -> Divide2/1
  Gain3/1 -> Divide2/2
  Selector/1 -> Diff Eta/1(SpdIn)

== system EvPowertrainController3EMDualFront/Energy Management/Control Domain /Rear Axle EM Torque Vector/3EM Dual Rear or 4EM ==
  EMAvgSpdVec : Inport
  Divide2 : Product  Inputs=**
  Dual EMs : Gain  Gain=2
  EMTrq Control Vector Traction : Constant  Value=linspace(0, max(PlntEM3Trq), CtrlVcuEMTrqSplitGrid)  SampleTime=-1
  Gain : Gain  Gain=-1
  Gain3 : Gain  Gain=PlntEMWhlGearRatioRL
  Gear Eta : Subsystem
  Selector : Selector  InputPortWidth=2  IndexOptions=Index vector (dialog)  Indices=[2]  OutputSizes=1
  WhlEMRearVecPos : Outport
  WhlEMRearVecNeg : Outport  Port=2
  wires:
  Gain3/1 -> Divide2/2
  EMAvgSpdVec/1 -> Selector/1
  EMTrq Control Vector Traction/1 -> Dual EMs/1
  Dual EMs/1 -> Gain3/1, Gear Eta/2(TrqIn)
  Gear Eta/1(eta) -> Divide2/1
  Divide2/1 -> Gain/1, WhlEMRearVecPos/1
  Gain/1 -> WhlEMRearVecNeg/1
  Selector/1 -> Gear Eta/1(SpdIn)

== system EvPowertrainController3EMDualFront/Energy Management/Convert Whl to EMTrq Vector/2EM/Diff Eta ==
  note: Pwr >= 0, v = 1
      | Pwr < 0, v= -1
  SpdIn : Inport
  TrqIn : Inport  Port=2
  Constant : Constant  Value=PlntDiffrntlEff
  Constant1 : Constant  SampleTime=-1
  Constant2 : Constant  Value=-1  SampleTime=-1
  Math Function1 : Math  Operator=pow  SignedPower=on  OutputSignalType=real
  Product1 : Product
  Switch2 : Switch  SaturateOnIntegerOverflow=off  InputSameDT=off
  eta : Outport  VectorParamsAs1DForOutWhenUnconnected=off
  wires:
  SpdIn/1 -> Product1/2
  Constant/1 -> Math Function1/1
  Constant2/1 -> Switch2/3
  Constant1/1 -> Switch2/1
  Product1/1 -> Switch2/2
  Switch2/1 -> Math Function1/2
  Math Function1/1 -> eta/1
  TrqIn/1 -> Product1/1

== system EvPowertrainController3EMDualFront/Energy Management/Convert Whl to EMTrq Vector/2EM/Diff Eta1 ==
  note: Pwr >= 0, v = 1
      | Pwr < 0, v= -1
  SpdIn : Inport
  TrqIn : Inport  Port=2
  Constant : Constant  Value=PlntDiffrntl2Eff
  Constant1 : Constant  SampleTime=-1
  Constant2 : Constant  Value=-1  SampleTime=-1
  Math Function1 : Math  Operator=pow  SignedPower=on  OutputSignalType=real
  Product1 : Product
  Switch2 : Switch  SaturateOnIntegerOverflow=off  InputSameDT=off
  eta : Outport  VectorParamsAs1DForOutWhenUnconnected=off
  wires:
  TrqIn/1 -> Product1/1
  Math Function1/1 -> eta/1
  Switch2/1 -> Math Function1/2
  Product1/1 -> Switch2/2
  Constant1/1 -> Switch2/1
  Constant2/1 -> Switch2/3
  Constant/1 -> Math Function1/1
  SpdIn/1 -> Product1/2

== system EvPowertrainController3EMDualFront/Energy Management/Convert Whl to EMTrq Vector/3EM Dual Front/Diff Eta ==
  note: Pwr >= 0, v = 1
      | Pwr < 0, v= -1
  SpdIn : Inport
  TrqIn : Inport  Port=2
  Constant : Constant  Value=PlntDiffrntl2Eff
  Constant1 : Constant  SampleTime=-1
  Constant2 : Constant  Value=-1  SampleTime=-1
  Math Function1 : Math  Operator=pow  SignedPower=on  OutputSignalType=real
  Product1 : Product
  Switch2 : Switch  SaturateOnIntegerOverflow=off  InputSameDT=off
  eta : Outport  VectorParamsAs1DForOutWhenUnconnected=off
  wires:
  SpdIn/1 -> Product1/2
  Constant/1 -> Math Function1/1
  Constant2/1 -> Switch2/3
  Constant1/1 -> Switch2/1
  Product1/1 -> Switch2/2
  Switch2/1 -> Math Function1/2
  Math Function1/1 -> eta/1
  TrqIn/1 -> Product1/1

== system EvPowertrainController3EMDualFront/Energy Management/Convert Whl to EMTrq Vector/3EM Dual Front/Gear Eta ==
  note: Pwr >= 0, v = 1
      | Pwr < 0, v= -1
  SpdIn : Inport
  TrqIn : Inport  Port=2
  Constant : Constant  Value=PlntEMWhlGearEffFL
  Constant1 : Constant  SampleTime=-1
  Constant2 : Constant  Value=-1  SampleTime=-1
  Math Function1 : Math  Operator=pow  SignedPower=on  OutputSignalType=real
  Product1 : Product
  Switch2 : Switch  SaturateOnIntegerOverflow=off  InputSameDT=off
  eta : Outport  VectorParamsAs1DForOutWhenUnconnected=off
  wires:
  TrqIn/1 -> Product1/1
  Math Function1/1 -> eta/1
  Switch2/1 -> Math Function1/2
  Product1/1 -> Switch2/2
  Constant1/1 -> Switch2/1
  Constant2/1 -> Switch2/3
  Constant/1 -> Math Function1/1
  SpdIn/1 -> Product1/2

== system EvPowertrainController3EMDualFront/Energy Management/Convert Whl to EMTrq Vector/3EM Dual Rear/Diff Eta ==
  note: Pwr >= 0, v = 1
      | Pwr < 0, v= -1
  SpdIn : Inport
  TrqIn : Inport  Port=2
  Constant : Constant  Value=PlntDiffrntlEff
  Constant1 : Constant  SampleTime=-1
  Constant2 : Constant  Value=-1  SampleTime=-1
  Math Function1 : Math  Operator=pow  SignedPower=on  OutputSignalType=real
  Product1 : Product
  Switch2 : Switch  SaturateOnIntegerOverflow=off  InputSameDT=off
  eta : Outport  VectorParamsAs1DForOutWhenUnconnected=off
  wires:
  SpdIn/1 -> Product1/2
  Constant/1 -> Math Function1/1
  Constant2/1 -> Switch2/3
  Constant1/1 -> Switch2/1
  Product1/1 -> Switch2/2
  Switch2/1 -> Math Function1/2
  Math Function1/1 -> eta/1
  TrqIn/1 -> Product1/1

== system EvPowertrainController3EMDualFront/Energy Management/Convert Whl to EMTrq Vector/3EM Dual Rear/Gear Eta ==
  note: Pwr >= 0, v = 1
      | Pwr < 0, v= -1
  SpdIn : Inport
  TrqIn : Inport  Port=2
  Constant : Constant  Value=PlntEMWhlGearEffRL
  Constant1 : Constant  SampleTime=-1
  Constant2 : Constant  Value=-1  SampleTime=-1
  Math Function1 : Math  Operator=pow  SignedPower=on  OutputSignalType=real
  Product1 : Product
  Switch2 : Switch  SaturateOnIntegerOverflow=off  InputSameDT=off
  eta : Outport  VectorParamsAs1DForOutWhenUnconnected=off
  wires:
  TrqIn/1 -> Product1/1
  Math Function1/1 -> eta/1
  Switch2/1 -> Math Function1/2
  Product1/1 -> Switch2/2
  Constant1/1 -> Switch2/1
  Constant2/1 -> Switch2/3
  Constant/1 -> Math Function1/1
  SpdIn/1 -> Product1/2

== system EvPowertrainController3EMDualFront/Energy Management/Convert Whl to EMTrq Vector/4EM/Gear Eta ==
  note: Pwr >= 0, v = 1
      | Pwr < 0, v= -1
  SpdIn : Inport
  TrqIn : Inport  Port=2
  Constant : Constant  Value=PlntEMWhlGearEffFL
  Constant1 : Constant  SampleTime=-1
  Constant2 : Constant  Value=-1  SampleTime=-1
  Math Function1 : Math  Operator=pow  SignedPower=on  OutputSignalType=real
  Product1 : Product
  Switch2 : Switch  SaturateOnIntegerOverflow=off  InputSameDT=off
  eta : Outport  VectorParamsAs1DForOutWhenUnconnected=off
  wires:
  TrqIn/1 -> Product1/1
  Math Function1/1 -> eta/1
  Switch2/1 -> Math Function1/2
  Product1/1 -> Switch2/2
  Constant1/1 -> Switch2/1
  Constant2/1 -> Switch2/3
  Constant/1 -> Math Function1/1
  SpdIn/1 -> Product1/2

== system EvPowertrainController3EMDualFront/Energy Management/Convert Whl to EMTrq Vector/4EM/Gear Eta1 ==
  note: Pwr >= 0, v = 1
      | Pwr < 0, v= -1
  SpdIn : Inport
  TrqIn : Inport  Port=2
  Constant : Constant  Value=PlntEMWhlGearEffRL
  Constant1 : Constant  SampleTime=-1
  Constant2 : Constant  Value=-1  SampleTime=-1
  Math Function1 : Math  Operator=pow  SignedPower=on  OutputSignalType=real
  Product1 : Product
  Switch2 : Switch  SaturateOnIntegerOverflow=off  InputSameDT=off
  eta : Outport  VectorParamsAs1DForOutWhenUnconnected=off
  wires:
  SpdIn/1 -> Product1/2
  Constant/1 -> Math Function1/1
  Constant2/1 -> Switch2/3
  Constant1/1 -> Switch2/1
  Product1/1 -> Switch2/2
  Switch2/1 -> Math Function1/2
  Math Function1/1 -> eta/1
  TrqIn/1 -> Product1/1

== system EvPowertrainController3EMDualFront/Energy Management/Powertrain Constraints /Battery Constraint/Electrical Current ==
  BattV : Inport
  EMPwrElecVec : Inport  Port=2
  DC-DC Eta : Subsystem  Variant=on  VariantControlMode=label  VariantControl=Variant1  LabelModeActiveChoice=0
  Divide : Product  Inputs=*/
  Saturation : Saturate  UpperLimit=Inf  LowerLimit=0.0001
  BatteryAmp : Outport  VectorParamsAs1DForOutWhenUnconnected=off
  wires:
  DC-DC Eta/1(Out) -> Divide/1
  EMPwrElecVec/1 -> DC-DC Eta/1(In)
  Divide/1 -> BatteryAmp/1
  BattV/1 -> Saturation/1
  Saturation/1 -> Divide/2

== system EvPowertrainController3EMDualFront/Energy Management/Powertrain Constraints /Battery Constraint/Power Limit Calculations ==
  note: Use Current Limits from BMS to calculate
      | discharge and charge power limits
  BattPwrDisChrgLmt : Inport
  "BattPwrChrgLmt " : Inport  Port=2
  BattV_in : Inport  Port=3
  Data Type Conversion : DataTypeConversion  SaturateOnIntegerOverflow=off  RndMeth=Floor
  Data Type Conversion1 : DataTypeConversion  SaturateOnIntegerOverflow=off  RndMeth=Floor
  Divide : Product  Inputs=*/
  Divide1 : Product  Inputs=/*
  div0protect - poly : autolibutils/div0protect - poly  thresh=.01  ZeroCross=off  ZeroCross1=on  aMode=aMode
  div0protect - poly1 : autolibutils/div0protect - poly  thresh=.01  ZeroCross=off  ZeroCross1=on  aMode=aMode
  BattCurrDischrgLmt : Outport  VectorParamsAs1DForOutWhenUnconnected=off
  BattCurrChrgLmt : Outport  Port=2  VectorParamsAs1DForOutWhenUnconnected=off
  BattPwrDischrgLmt : Outport  Port=3  VectorParamsAs1DForOutWhenUnconnected=off
  BattPwrChrgLmt : Outport  Port=4  VectorParamsAs1DForOutWhenUnconnected=off
  wires:
  "BattPwrChrgLmt "/1 -> Divide1/2, Data Type Conversion/1
  BattPwrDisChrgLmt/1 -> Divide/1, Data Type Conversion1/1
  Data Type Conversion/1 -> BattPwrChrgLmt/1
  Data Type Conversion1/1 -> BattPwrDischrgLmt/1
  Divide/1 -> BattCurrDischrgLmt/1
  BattV_in/1 -> div0protect - poly/1, div0protect - poly1/1
  Divide1/1 -> BattCurrChrgLmt/1
  div0protect - poly/1 -> Divide1/1
  div0protect - poly1/1 -> Divide/2

== system EvPowertrainController3EMDualFront/Energy Management/Powertrain Constraints /EM Constraint Front/Maximum Torque ==
  note: Don't allow negative MotTrq when
      | WhlTrqCmd is >= 0
  WhlTrqCmd : Inport
  WhlEMTrqSplitVecFrnt : Inport  Port=2
  WhlTrqMaxVec : Inport  Port=3
  Compare To Zero : simulink/Logic and Bit Operations/Compare To Zero  relop=<  OutDataTypeStr=boolean
  Compare To Zero1 : simulink/Logic and Bit Operations/Compare To Zero  relop=>=  OutDataTypeStr=boolean
  Gain : Gain  Gain=-1
  Logical Operator : Logic  Operator=OR  Inputs=3  AllPortsSameDT=off  OutDataTypeStr=boolean
  Logical Operator1 : Logic  AllPortsSameDT=off  OutDataTypeStr=boolean
  Relational Operator : RelationalOperator  Operator=<  OutDataTypeStr=boolean  RndMeth=Simplest  InputSameDT=off
  Relational Operator1 : RelationalOperator  Operator=<  OutDataTypeStr=boolean  RndMeth=Simplest  InputSameDT=off
  Saturation Dynamic : simulink/Discontinuities/Saturation Dynamic  OutMin=[]  OutMax=[]  OutDataTypeStr=Inherit: Same as second input  OutDataType=fixdt(1, 16)  OutScaling=2^-10  DoSatur=off
  WhlEMTrqSatVec : Outport  VectorParamsAs1DForOutWhenUnconnected=off
  InfeasibleEMVec : Outport  Port=2  VectorParamsAs1DForOutWhenUnconnected=off
  wires:
  Logical Operator1/1 -> Logical Operator/3
  Compare To Zero1/1 -> Logical Operator1/2
  WhlEMTrqSplitVecFrnt/1 -> Relational Operator/2, Relational Operator1/1, Saturation Dynamic/2, Compare To Zero/1
  Compare To Zero/1 -> Logical Operator1/1
  WhlTrqCmd/1 -> Compare To Zero1/1
  Gain/1 -> Relational Operator1/2, Saturation Dynamic/3
  Saturation Dynamic/1 -> WhlEMTrqSatVec/1
  Relational Operator/1 -> Logical Operator/1
  Relational Operator1/1 -> Logical Operator/2
  Logical Operator/1 -> InfeasibleEMVec/1
  WhlTrqMaxVec/1 -> Gain/1, Relational Operator/1, Saturation Dynamic/1

== system EvPowertrainController3EMDualFront/Energy Management/Powertrain Constraints /EM Constraint Front/Tabular Power Loss Data ==
  EMAvgSpdVec : Inport
  WhlEMTrqSatVec : Inport  Port=2
  2EM or 3EM Dual Rear : Subsystem  VariantControl=2EM or 3EM Dual Rear
  3EM Dual Front or 4EM : Subsystem  VariantControl=3EM Dual Front or 4EM
  EMPwrElecVec : Outport

== system EvPowertrainController3EMDualFront/Energy Management/Powertrain Constraints /EM Constraint Rear/Maximum Torque ==
  note: Don't allow negative MotTrq when
      | WhlTrqCmd is >= 0
  WhlTrqCmd : Inport
  WhlEMTrqSplitVecRear : Inport  Port=2
  WhlTrqMaxVec : Inport  Port=3
  Compare To Zero : simulink/Logic and Bit Operations/Compare To Zero  relop=<  OutDataTypeStr=boolean
  Compare To Zero1 : simulink/Logic and Bit Operations/Compare To Zero  relop=>=  OutDataTypeStr=boolean
  Gain : Gain  Gain=-1
  Logical Operator : Logic  Operator=OR  Inputs=3  AllPortsSameDT=off  OutDataTypeStr=boolean
  Logical Operator1 : Logic  AllPortsSameDT=off  OutDataTypeStr=boolean
  Relational Operator : RelationalOperator  Operator=<  OutDataTypeStr=boolean  RndMeth=Simplest  InputSameDT=off
  Relational Operator1 : RelationalOperator  Operator=<  OutDataTypeStr=boolean  RndMeth=Simplest  InputSameDT=off
  Saturation Dynamic : simulink/Discontinuities/Saturation Dynamic  OutMin=[]  OutMax=[]  OutDataTypeStr=Inherit: Same as second input  OutDataType=fixdt(1, 16)  OutScaling=2^-10  DoSatur=off
  WhlEMTrqSatVec : Outport  VectorParamsAs1DForOutWhenUnconnected=off
  InfeasibleEMVec : Outport  Port=2  VectorParamsAs1DForOutWhenUnconnected=off
  wires:
  WhlTrqMaxVec/1 -> Saturation Dynamic/1, Relational Operator/1, Gain/1
  Logical Operator/1 -> InfeasibleEMVec/1
  Relational Operator1/1 -> Logical Operator/2
  Relational Operator/1 -> Logical Operator/1
  Saturation Dynamic/1 -> WhlEMTrqSatVec/1
  Gain/1 -> Saturation Dynamic/3, Relational Operator1/2
  WhlTrqCmd/1 -> Compare To Zero1/1
  Compare To Zero/1 -> Logical Operator1/1
  WhlEMTrqSplitVecRear/1 -> Compare To Zero/1, Saturation Dynamic/2, Relational Operator1/1, Relational Operator/2
  Compare To Zero1/1 -> Logical Operator1/2
  Logical Operator1/1 -> Logical Operator/3

== system EvPowertrainController3EMDualFront/Energy Management/Powertrain Constraints /EM Constraint Rear/Tabular Power Loss Data ==
  EMAvgSpdVec : Inport
  WhlEMTrqSatVec : Inport  Port=2
  2EM : Subsystem  VariantControl=2EM
  3EM Dual Front : Subsystem  VariantControl=3EM Dual Front
  3EM Dual Rear or 4EM : Subsystem  VariantControl=3EM Dual Rear or 4EM
  EMPwrElecVec : Outport

== system EvPowertrainController3EMDualFront/Torque Vectoring/3EM/Create EMTrq Vector/3EMDualFront ==
  EMTrqSplit : Inport
  EMTrqCmd : Inport  Port=2
  Selector : Selector  InputPortWidth=3  IndexOptions=Index vector (dialog)  Indices=[3]  OutputSizes=1
  Vector Concatenate : Concatenate
  EMTrqCmdFinal : Outport
  wires:
  Selector/1 -> Vector Concatenate/2
  EMTrqCmd/1 -> Selector/1
  Vector Concatenate/1 -> EMTrqCmdFinal/1
  EMTrqSplit/1 -> Vector Concatenate/1

== system EvPowertrainController3EMDualFront/Torque Vectoring/3EM/Create EMTrq Vector/3EMDualRear ==
  EMTrqSplit : Inport
  EMTrqCmd : Inport  Port=2
  Selector : Selector  InputPortWidth=3  IndexOptions=Index vector (dialog)  Indices=[1]  OutputSizes=1
  Vector Concatenate : Concatenate
  EMTrqCmdFinal : Outport
  wires:
  Selector/1 -> Vector Concatenate/1
  EMTrqSplit/1 -> Vector Concatenate/2
  Vector Concatenate/1 -> EMTrqCmdFinal/1
  EMTrqCmd/1 -> Selector/1

== system EvPowertrainController3EMDualFront/Torque Vectoring/3EM/EMTrq/3EMDualFront ==
  EMSpd : Inport
  EMTrqCmd : Inport  Port=2
  1-D Lookup Table : Lookup_n-D  NumberOfTableDimensions=1  BreakpointsForDimension1=PlntEM3Spd  Table=PlntEM3Trq  ExtrapMethod=Clip  UseLastTableValue=on  InternalRulePriority=Speed  RndMeth=Simplest
  3EMDualFront : Subsystem  VariantControl=3EMDualFront
  Abs1 : Abs  SaturateOnIntegerOverflow=off
  Selector : Selector  InputPortWidth=3  IndexOptions=Index vector (dialog)  Indices=[1]  OutputSizes=1
  Selector1 : Selector  InputPortWidth=3  IndexOptions=Index vector (dialog)  Indices=[2]  OutputSizes=1
  EMTrqMax : Outport
  EMTrqL : Outport  Port=2
  EMTrqR : Outport  Port=3
  wires:
  Selector1/1 -> EMTrqR/1
  Selector/1 -> EMTrqL/1
  EMTrqCmd/1 -> Selector/1, Selector1/1
  3EMDualFront/1(EMSpdAvg) -> Abs1/1
  1-D Lookup Table/1 -> EMTrqMax/1
  EMSpd/1 -> 3EMDualFront/1(EMSpd)
  Abs1/1 -> 1-D Lookup Table/1

== system EvPowertrainController3EMDualFront/Torque Vectoring/3EM/EMTrq/3EMDualRear ==
  EMSpd : Inport
  EMTrqCmd : Inport  Port=2
  1-D Lookup Table : Lookup_n-D  NumberOfTableDimensions=1  BreakpointsForDimension1=PlntEM3Spd  Table=PlntEM3Trq  ExtrapMethod=Clip  UseLastTableValue=on  InternalRulePriority=Speed  RndMeth=Simplest
  3EMDualRear : Subsystem  VariantControl=3EMDualRear
  Abs1 : Abs  SaturateOnIntegerOverflow=off
  Selector : Selector  InputPortWidth=3  IndexOptions=Index vector (dialog)  Indices=[2]  OutputSizes=1
  Selector1 : Selector  InputPortWidth=3  IndexOptions=Index vector (dialog)  Indices=[3]  OutputSizes=1
  EMTrqMax : Outport
  EMTrqL : Outport  Port=2
  EMTrqR : Outport  Port=3
  wires:
  EMTrqCmd/1 -> Selector/1, Selector1/1
  Selector/1 -> EMTrqL/1
  Selector1/1 -> EMTrqR/1
  Abs1/1 -> 1-D Lookup Table/1
  EMSpd/1 -> 3EMDualRear/1(EMSpd)
  1-D Lookup Table/1 -> EMTrqMax/1
  3EMDualRear/1(EMSpdAvg) -> Abs1/1
